simulink model "lv_Cp"  (Simulink 7.1)
settings: Solver=ode45  StartTime=0.0  StopTime=100  RelTol=1e-3
values from neighbouring files (symbols this model uses):
  C1 = 0.44    [lv_demofile.m]    (also in lv_demofile1.m; lv_demofile2.m; lv_demofile4.m; lv_demofile5.m)
  C2 = 0.0167    [lv_demofile.m]    (also in lv_demofile1.m; lv_demofile2.m; lv_demofile4.m; lv_demofile5.m)
  C3 = 0.3    [lv_demofile.m]    (also in lv_demofile1.m; lv_demofile2.m; lv_demofile4.m; lv_demofile5.m)
  C4 = 0.00184    [lv_demofile.m]    (also in lv_demofile1.m; lv_demofile2.m; lv_demofile4.m; lv_demofile5.m)
settings Model: Creator=lv  LastModifiedBy=lv

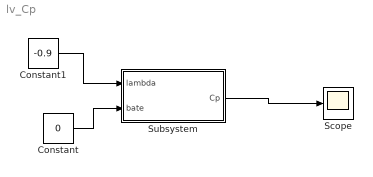
== system lv_Cp ==
  Constant : Constant  Value=0  OutDataType=sfix(16)  OutScaling=2^0
  Constant1 : Constant  Value=-0.9  OutDataType=sfix(16)  OutScaling=2^0
  Scope : Scope
  Subsystem : Subsystem
  wires:
  Constant1/1 -> Subsystem/1(lambda)
  Constant/1 -> Subsystem/2(bate)
  Subsystem/1(Cp) -> Scope/1

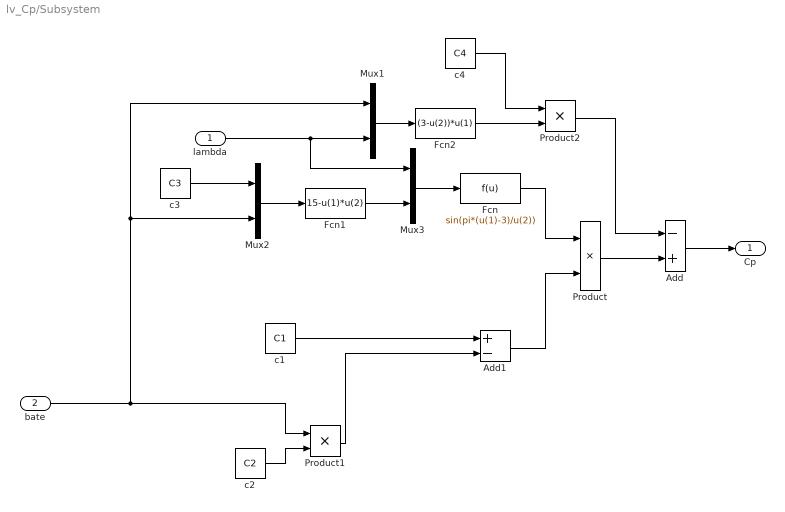
== system lv_Cp/Subsystem ==
  lambda : Inport  OutDataType=sfix(16)  OutScaling=2^0
  bate : Inport  Port=2  OutDataType=sfix(16)  OutScaling=2^0
  Add : Sum  Inputs=-+  OutDataType=sfix(16)  OutScaling=2^-10
  Add1 : Sum  Inputs=+-  OutDataType=sfix(16)  OutScaling=2^-10
  Fcn : Fcn  Expr=sin(pi*(u(1)-3)/u(2))
  Fcn1 : Fcn  Expr=15-u(1)*u(2)
  Fcn2 : Fcn  Expr=(3-u(2))*u(1)
  Mux1 : Mux  Inputs=2
  Mux2 : Mux  Inputs=2
  Mux3 : Mux  Inputs=2
  Product : Product  OutDataType=sfix(16)  OutScaling=2^0  RndMeth=Zero
  Product1 : Product  OutDataType=sfix(16)  OutScaling=2^0  RndMeth=Zero
  Product2 : Product  OutDataType=sfix(16)  OutScaling=2^0  RndMeth=Zero
  c1 : Constant  Value=C1  OutDataType=sfix(16)  OutScaling=2^0
  c2 : Constant  Value=C2  OutDataType=sfix(16)  OutScaling=2^0
  c3 : Constant  Value=C3  OutDataType=sfix(16)  OutScaling=2^0
  c4 : Constant  Value=C4  OutDataType=sfix(16)  OutScaling=2^0
  Cp : Outport  OutDataType=sfix(16)  OutScaling=2^0
  wires:
  c1/1 -> Add1/1
  bate/1 -> Product1/1, Mux2/2, Mux1/1
  c2/1 -> Product1/2
  Product1/1 -> Add1/2
  Mux2/1 -> Fcn1/1
  c3/1 -> Mux2/1
  Mux3/1 -> Fcn/1
  Fcn/1 -> Product/1
  Add1/1 -> Product/2
  Product/1 -> Add/2
  Fcn1/1 -> Mux3/2
  lambda/1 -> Mux3/1, Mux1/2
  Mux1/1 -> Fcn2/1
  c4/1 -> Product2/1
  Fcn2/1 -> Product2/2
  Product2/1 -> Add/1
  Add/1 -> Cp/1
